simulink model "CalculatorRoot"  (Simulink 8.7)
settings: Solver=ode45  StartTime=0.0  StopTime=10.0  RelTol=1e-3
PreLoadFcn:
  | addpath ('../ProcAbs');
  | addpath ('../ProcAdd');
  | addpath ('../Divide');
  | addpath('../Utilities');
  | addpath('./scripts');
  | addpath ('../../../parameters');
PostSaveFcn:
  | CallBack
  | Generate
  | Setup
CloseFcn:
  | callback1
  | callback2
  | param1
settings Model: Creator=PLM\yymatlab  LastModifiedBy=PLM\cuo1oa
settings DataIOCC: SignalLoggingSaveFormat=ModelDataLogs
settings OptimizationCC: ExpressionDepthLimit=2147483647
settings DebuggingCC: SolverPrmCheckMsg=warning  FcnCallInpInsideContextMsg=EnableAllAsWarning  StateNameClashWarn=warning
settings GRTTargetCC: CombineOutputUpdateFcns=off  GRTInterface=on
settings ConfigComp: CovSFcnEnable=off

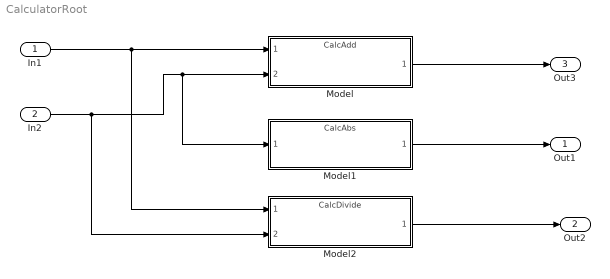
== system CalculatorRoot ==
  In1 : Inport
  In2 : Inport  Port=2
  Model : ModelReference  ModelNameDialog=CalcAdd  SimulationMode=Normal  ModelReferenceVersion=1.5
  Model1 : ModelReference  ModelNameDialog=CalcAbs  SimulationMode=Normal  ModelReferenceVersion=1.4
  Model2 : ModelReference  ModelNameDialog=CalcDivide  SimulationMode=Normal  ModelReferenceVersion=1.4
  Out1 : Outport
  Out2 : Outport  Port=2
  Out3 : Outport  Port=3
  wires:
  In1/1 -> Model2/1, Model/1
  In2/1 -> Model2/2, Model1/1, Model/2
  Model/1 -> Out3/1
  Model1/1 -> Out1/1
  Model2/1 -> Out2/1
